simulink model "DCMotorModel"  (R2025b)
settings: Solver=VariableStepAuto  StartTime=0.0  StopTime=10  FixedStep=0.1  RelTol=1e-3
libraries: slpidlib x1, simulink x1
settings Model: Creator=nps22  LastModifiedBy=jujma

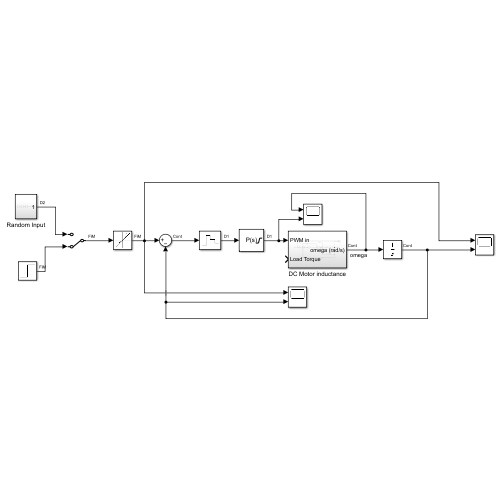
[thumbnail: Simulink's stored preview of the top-level diagram]
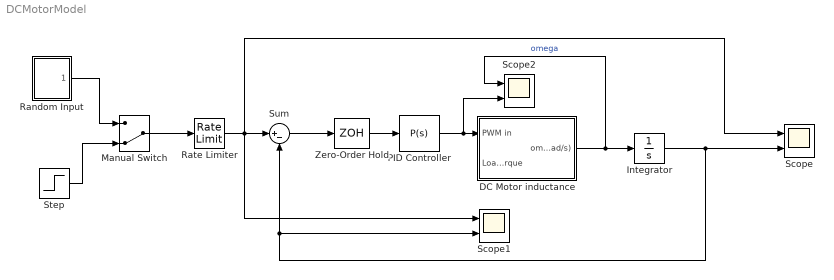
== system DCMotorModel ==
  DC Motor inductance : Subsystem
  Integrator : Integrator
  Manual Switch : ManualSwitch  CurrentSetting=0
  PID Controller : slpidlib/PID Controller  Controller=P  Form=Parallel  TimeDomain=Continuous-time  UseExternalTs=off  SampleTime=-1  IntegratorMethod=Forward Euler  FilterMethod=Forward Euler  ControllerParametersSource=internal  P=0.01  I=1  UseKiTs=off  D=0  UseExternalDerivativeSource=off  N=100  UseFilter=on  TunerSelectOption=Transfer Function Based (PID Tuner App)  InitialConditionSource=internal  InitialConditionForIntegrator=0  InitialConditionForFilter=0  DifferentiatorICPrevScaledInput=0  ExternalReset=none  TrackingMode=off  Kt=1  LimitOutput=on  SatLimitsSource=internal  UpperSaturationLimit=1  LowerSaturationLimit=-1  LinearizeAsGain=on  AntiWindupMode=none  Kb=1  LimitIntegrator=off  UpperIntegratorSaturationLimit=inf  LowerIntegratorSaturationLimit=-inf  POutMin=[]  POutMax=[]  IOutMin=[]  IOutMax=[]  DOutMin=[]  DOutMax=[]  NOutMin=[]  NOutMax=[]  SumOutMin=[]  SumOutMax=[]  SaturationOutMin=[]  SaturationOutMax=[]  PParamMin=[]  PParamMax=[]  IParamMin=[]  IParamMax=[]  DParamMin=[]  DParamMax=[]  NParamMin=[]  NParamMax=[]  KbParamMin=[]  KbParamMax=[]  KtParamMin=[]  KtParamMax=[]  KbOutMin=[]  KbOutMax=[]  KtOutMin=[]  KtOutMax=[]  IntegratorOutMin=[]  IntegratorOutMax=[]  FilterOutMin=[]  FilterOutMax=[]  SumI1OutMin=[]  SumI1OutMax=[]  SumI2OutMin=[]  SumI2OutMax=[]  SumI3OutMin=[]  SumI3OutMax=[]  SumI4OutMin=[]  SumI4OutMax=[]  SumDOutMin=[]  SumDOutMax=[]  DifferentiatorOutMin=[]  DifferentiatorOutMax=[]  FilterDiffOutCoefMin=[]  FilterDiffOutCoefMax=[]  ReciprocalOutMin=[]  ReciprocalOutMax=[]  SumDenOutMin=[]  SumDenOutMax=[]  SumNumOutMin=[]  SumNumOutMax=[]  DivideOutMin=[]  DivideOutMax=[]  UdiffTsProdOutMin=[]  UdiffTsProdOutMax=[]  NTsProdOutMin=[]  NTsProdOutMax=[]  UintegralTsProdOutMin=[]  UintegralTsProdOutMax=[]  UngainTsProdOutMin=[]  UngainTsProdOutMax=[]  ClampingZeroOutDataTypeStr=Inherit: Inherit via back propagation  ClampingZeroOutMin=[]  ClampingZeroOutMax=[]  FilterDenConstantOutDataTypeStr=Inherit: Inherit via back propagation  FilterDenConstantOutMin=[]  FilterDenConstantOutMax=[]  PCopyOutDataTypeStr=Inherit: Inherit via back propagation  PCopyOutMin=[]  PCopyOutMax=[]  NCopyOutDataTypeStr=Inherit: Inherit via back propagation  NCopyOutMin=[]  NCopyOutMax=[]  IntegratorContinuousStateAttributes=''  IntegratorStateMustResolveToSignalObject=off  IntegratorRTWStateStorageClass=Auto  FilterContinuousStateAttributes=''  FilterStateMustResolveToSignalObject=off  FilterRTWStateStorageClass=Auto  ParallelPVariant=InternalParameters  IdealPVariant=Disabled  IVariant=Disabled  DVariant=Disabled  IntegratorVariant=Disabled  SatVariant=Enabled  AWVariant=Disabled  PCopyVariant=Disabled  TRVariant=Disabled  FdbkBlocksVariant=Forward  IdealPFdbkVariant=Disabled  SatFdbkVariant=Disabled  DerivativeFilterVariant=Disabled  NVariant=Disabled  NCopyVariant=Disabled_SignalSpec  FilterICVariant=Disabled  IntegratorICVariant=Disabled  ExternalResetVariant=Disabled  TRSumVariant=Passthrough  SumFdbkVariant=Disabled  SumVariant=Passthrough_P  TsampFilterVariant=InternalTs  TsampNgainVariant=Passthrough  TsampIntegralVariant=Disabled_SignalSpec  ExternalSaturationOutDataTypeStr=Inherit: Same as second input  DerivativeSourceVariant=Disabled  PreIntVariant=InternalPreInt
  Random Input : Subsystem
  Rate Limiter : RateLimiter  RisingSlewLimit=500  FallingSlewLimit=-500  SampleTimeMode=inherited
  Scope : Scope  NumInputPorts=2
      settings: ActiveDisplayYMinimum=-125.00000005212179  ActiveDisplayYMaximum=1125.0000004689507
  Scope1 : Scope  NumInputPorts=2
      settings: ActiveDisplayYMinimum=-124.99999999999997  ActiveDisplayYMaximum=1125  DataLoggingVariableName=ScopeData2
  Scope2 : Scope  NumInputPorts=2
      settings: ActiveDisplayYMinimum=283.88373980455344  ActiveDisplayYMaximum=538.39324107696757
  Step : Step  After=1000  SampleTime=0
  Sum : Sum  Inputs=|+-
  Zero-Order Hold : ZeroOrderHold  SampleTime=0.1
  wires:
  DC Motor inductance/1(omega (rad/s)) -> Scope2/1, Integrator/1  "omega"
  Manual Switch/1 -> Rate Limiter/1
  Random Input/1(Out1) -> Manual Switch/1
  Step/1 -> Manual Switch/2
  PID Controller/1 -> Scope2/2, DC Motor inductance/1(PWM in)
  Integrator/1 -> Scope1/2, Sum/2, Scope/2
  Rate Limiter/1 -> Scope1/1, Scope/1, Sum/1
  Zero-Order Hold/1 -> PID Controller/1
  Sum/1 -> Zero-Order Hold/1

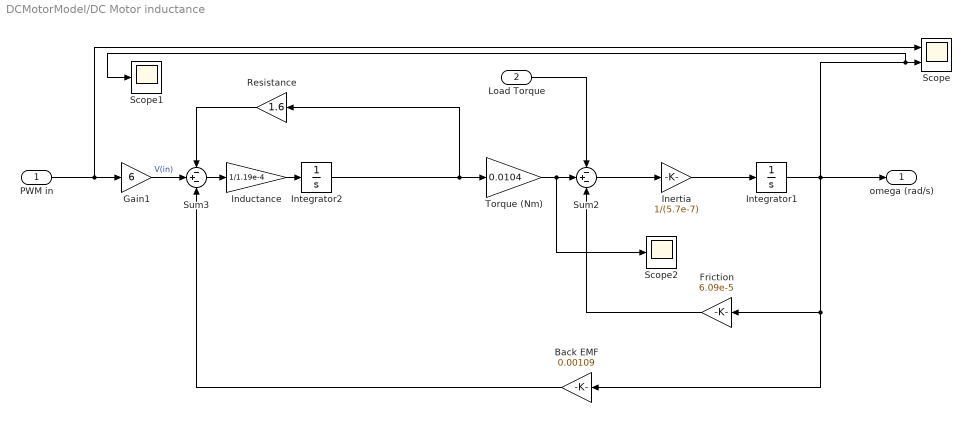
== system DCMotorModel/DC Motor inductance ==
  PWM in : Inport
  Load Torque : Inport  Port=2
  Back EMF : Gain  Gain=0.00109
  Friction : Gain  Gain=6.09e-5
  Gain1 : Gain  Gain=6
  Inductance : Gain  Gain=1/1.19e-4
  Inertia : Gain  Gain=1/(5.7e-7)
  Integrator1 : Integrator
  Integrator2 : Integrator
  Resistance : Gain  Gain=1.6
  Scope : Scope  NumInputPorts=2
      settings: ActiveDisplayYMinimum=-0.12500005559101079  ActiveDisplayYMaximum=1.1250000061767791
  Scope1 : Scope
      settings: DataLoggingVariableName=ScopeData3
  Scope2 : Scope
      settings: ActiveDisplayYMinimum=-0.0048479602001581046  ActiveDisplayYMaximum=0.043631641801422948
  Sum2 : Sum  Inputs=-+-
  Sum3 : Sum  Inputs=-+-
  Torque (Nm) : Gain  Gain=0.0104
  omega (rad/s) : Outport
  wires:
  Back EMF/1 -> Sum3/3
  Resistance/1 -> Sum3/1
  Inertia/1 -> Integrator1/1
  Sum3/1 -> Inductance/1
  Friction/1 -> Sum2/3
  Sum2/1 -> Inertia/1
  Integrator1/1 -> Scope1/1, Scope/2, omega (rad/s)/1, Friction/1, Back EMF/1
  Inductance/1 -> Integrator2/1
  Torque (Nm)/1 -> Scope2/1, Sum2/2
  Load Torque/1 -> Sum2/1
  Gain1/1 -> Sum3/2  "V(in)"
  PWM in/1 -> Scope/1, Gain1/1
  Integrator2/1 -> Resistance/1, Torque (Nm)/1

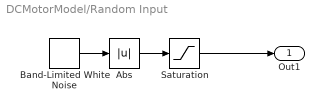
== system DCMotorModel/Random Input ==
  Abs : Abs  SaturateOnIntegerOverflow=off
  Band-Limited White Noise : simulink/Sources/Band-Limited White Noise  Cov=[3e4]  Ts=1  seed=[23341]
  Saturation : Saturate  UpperLimit=350  LowerLimit=0
  Out1 : Outport
  wires:
  Abs/1 -> Saturation/1
  Band-Limited White Noise/1 -> Abs/1
  Saturation/1 -> Out1/1
